simulink model "untitled1"  (R2017a)
settings: Solver=VariableStepAuto  StartTime=0.0  StopTime=10.0  RelTol=1e-3
settings Model: Creator=misbah  LastModifiedBy=misbah

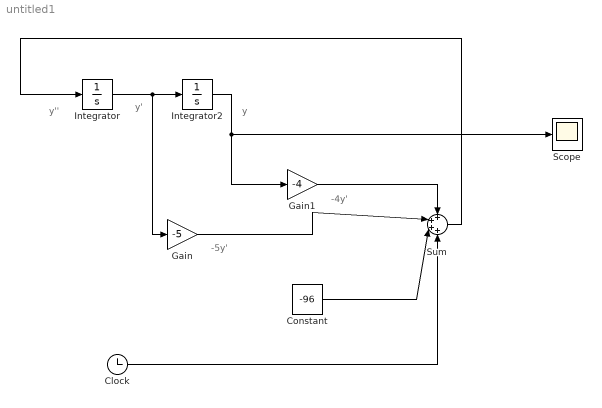
== system untitled1 ==
  note: -4y'
  note: -5y'
  note: y
  note: y'
  note: y''
  Clock : Clock
  Constant : Constant  Value=-96
  Gain : Gain  Gain=-5
  Gain1 : Gain  Gain=-4
  Integrator : Integrator  InitialCondition=16
  Integrator2 : Integrator  InitialCondition=4
  Scope : Scope
  Sum : Sum  Inputs=++++
  wires:
  Integrator/1 -> Gain/1, Integrator2/1
  Integrator2/1 -> Scope/1, Gain1/1
  Gain/1 -> Sum/2
  Gain1/1 -> Sum/1
  Constant/1 -> Sum/3
  Sum/1 -> Integrator/1
  Clock/1 -> Sum/4
